simulink model "set_sas"  (R2020a)
settings: Solver=FixedStepDiscrete  StartTime=0.0  StopTime=10.0  RelTol=1e-3
settings Model: Creator=thomas  LastModifiedBy=thomas

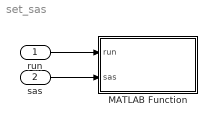
== system set_sas ==
  run : Inport  OutDataTypeStr=boolean
  sas : Inport  Port=2  OutDataTypeStr=boolean
  MATLAB Function : MATLAB Function  TreatAsAtomicUnit=on
  wires:
  sas/1 -> MATLAB Function/2(sas)
  run/1 -> MATLAB Function/1(run)

== matlab function set_sas/MATLAB Function ==
  data: run input; sas input boolean
function set_sas(run, sas)
    coder.extrinsic('evalin');
    if run
        evalin('base', sprintf('vessel_control.setSAS(%u);', uint8(sas)));
    end
end
